simulink model "aeration_system"  (R2023a)
settings: Solver=FixedStepAuto  StartTime=0.0  StopTime=10.0  FixedStep=0.1  RelTol=1e-3
settings Model: Creator=Lucca  LastModifiedBy=Lucca

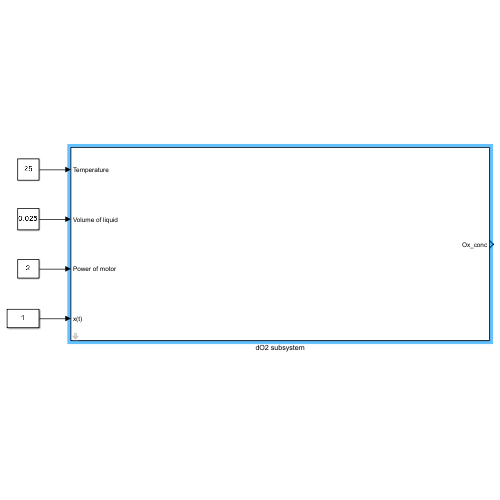
[thumbnail: Simulink's stored preview of the top-level diagram]
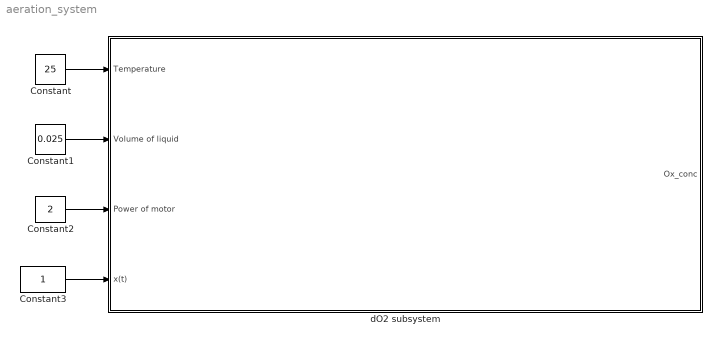
== system aeration_system ==
  Constant : Constant  Value=25
  Constant1 : Constant  Value=0.025
  Constant2 : Constant  Value=2
  Constant3 : Constant
  dO2 subsystem : Subsystem  mask{Air_flow=0.0001, r=0.00125, d=0.0025, viscosity=0.001, O_consumed=0.0001, Ti=25, A=750, C=0.026, alpha=0.4, beta=0.5, delta=0.55, m=-0.1446, e=11.999}
      mask prompts: Air_flow "air flow (m^3 /s)"; r "radius of vessel (m)"; d "diameter of impeller (m)"; viscosity "viscosity (Pa*s)"; O_consumed "Oxygen consumed per mass of biomass (mg/s)"; Ti "initial temperature (deg C)"; A "constant 1 (A)"; C "constant 2 (C)"; alpha "constant 3 (alpha)"; beta "constant 4 (beta)"; delta "constant 5 (delta)"; m "constant 6 (m)"; e "constant 7 (c)"
  wires:
  Constant/1 -> dO2 subsystem/1(Temperature)
  Constant1/1 -> dO2 subsystem/2(Volume of liquid)
  Constant2/1 -> dO2 subsystem/3(Power of motor)
  Constant3/1 -> dO2 subsystem/4(x(t))

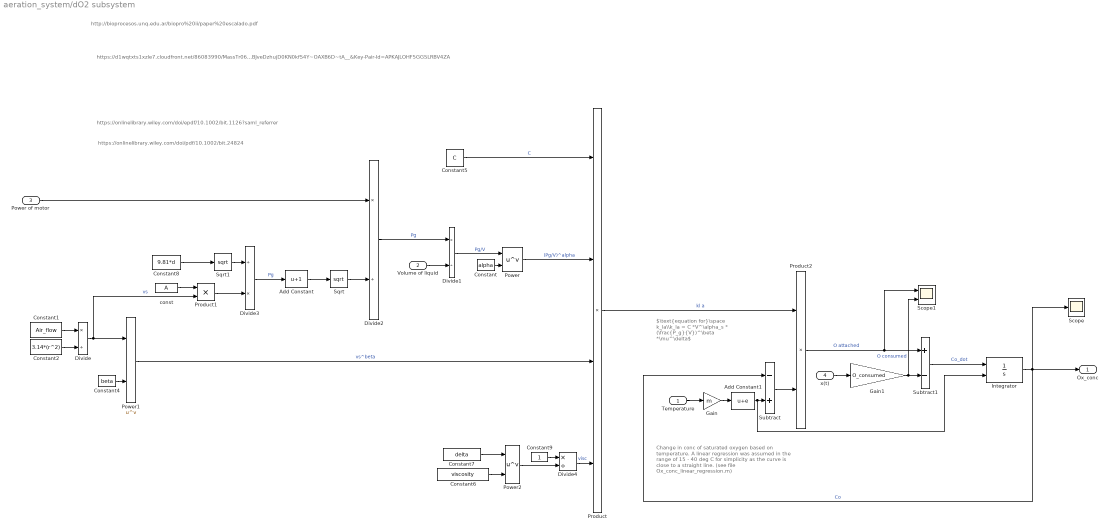
== system aeration_system/dO2 subsystem ==
  note: Change in conc of saturated oxygen based on temperature. A linear regression was assumed in the range of 15 - 40 deg C for simplicity as the curve is close to a straight line. (see file Ox_conc_linear_regression.m)
  note: $\text{equation for}\space k_la\\k_la = C *V^\alpha_s * (\frac{P_g}{V})^\beta *\mu^\delta$
  note: http://bioprocesos.unq.edu.ar/biopro%20ii/paper%20escalado.pdf
  note: https://d1wqtxts1xzle7.cloudfront.net/86083990/MassTr06-libre.pdf?1652828187=&response-content-disposition=inline%3B+filename%3DSimultaneous_Determination_of_Oxygen_Con.pdf&Expires=1693320232&Signature=cT0WufUoFrxjuPdJGbVLo4QoXSVqB1llCupeDkbPwvBGTrAJrYMzSobRzxnkgx671FYnx4G-HWNW9pRr5rOW2sojiWm9-xMMdIoObZIgvwRAe8ddChCfE4EtN7E38vVW-~N8isqnocr2KooJIBzTXSX1d969dYKALbyDclzDGhk2mnBZWyIczpO0KS24b7NT1cVUENKGDnwmfNy8UIRDn-Ug2fUkbjvOlAl2LNzg1gb-glHg-VDiAp-56qrcyUVPospzmfTVz7spUSZfQoSY3Tq-v9C5ADxviKRit4iZjO~6Dx7r1IDkGxiLGBJveDzhujD0KN0kfS4Y~OAXB6D~tA__&Key-Pair-Id=APKAJLOHF5GGSLRBV4ZA
  note: https://onlinelibrary.wiley.com/doi/pdf/10.1002/bit.24824
  note: https://onlinelibrary.wiley.com/doi/epdf/10.1002/bit.1126?saml_referrer
  Temperature : Inport
  Volume of liquid : Inport  Port=2
  Power of motor : Inport  Port=3
  x(t) : Inport  Port=4
  Add Constant : Bias  Bias=1  SaturateOnIntegerOverflow=off
  Add Constant1 : Bias  Bias=e  SaturateOnIntegerOverflow=off
  Constant : Constant  Value=alpha
  Constant1 : Constant  Value=Air_flow
  Constant2 : Constant  Value=3.14*(r^2)
  Constant4 : Constant  Value=beta
  Constant5 : Constant  Value=C
  Constant6 : Constant  Value=viscosity
  Constant7 : Constant  Value=delta
  Constant8 : Constant  Value=9.81*d
  Constant9 : Constant
  Divide{,1..2,4} (4 alike) : Product  Inputs=*/
  Divide3 : Product  Inputs=/*
  Gain : Gain  Gain=m
  Gain1 : Gain  Gain=O_consumed
  Integrator : Integrator  InitialConditionSource=external  InitialCondition=m*Ti + e
  Power : Math  Operator=pow
  Power1 : Math  Operator=pow
  Power2 : Math  Operator=pow
  Product : Product  Inputs=4
  Product1 : Product
  Product2 : Product
  Scope : Scope
  Scope1 : Scope  NumInputPorts=2
  Sqrt : Sqrt
  Sqrt1 : Sqrt
  Subtract : Sum  Inputs=-+
  Subtract1 : Sum  Inputs=+-
  const : Constant  Value=A
  Ox_conc : Outport
  wires:
  Power/1 -> Product/2  "(Pg/V)^alpha"
  Product1/1 -> Divide3/2
  Divide/1 -> Power1/1, Product1/2  "vs"
  const/1 -> Product1/1
  Constant4/1 -> Power1/2
  Add Constant/1 -> Sqrt/1
  Product/1 -> Product2/1  "kl a"
  Constant5/1 -> Product/1  "C"
  Power1/1 -> Product/3  "vs^beta"
  Divide3/1 -> Add Constant/1  "Pg"
  Sqrt1/1 -> Divide3/1
  Constant1/1 -> Divide/1
  Constant/1 -> Power/2
  Constant8/1 -> Sqrt1/1
  Divide1/1 -> Power/1  "Pg/V"
  Power2/1 -> Divide4/2
  Constant7/1 -> Power2/1
  Constant6/1 -> Power2/2
  Constant2/1 -> Divide/2
  Volume of liquid/1 -> Divide1/2
  Divide2/1 -> Divide1/1  "Pg"
  Power of motor/1 -> Divide2/1
  Subtract1/1 -> Integrator/1  "Co_dot"
  Integrator/1 -> Ox_conc/1, Scope/1, Subtract/1  "Co"
  Temperature/1 -> Gain/1
  Gain/1 -> Add Constant1/1
  Add Constant1/1 -> Integrator/2, Subtract/2
  Subtract/1 -> Product2/2
  Product2/1 -> Scope1/1, Subtract1/1  "O attached"
  x(t)/1 -> Gain1/1
  Gain1/1 -> Scope1/2, Subtract1/2  "O consumed"
  Sqrt/1 -> Divide2/2
  Constant9/1 -> Divide4/1
  Divide4/1 -> Product/4  "visc"
